simulink model "EM_SS_Model"  (R2017b)
settings: Solver=VariableStepAuto  StartTime=0.0  StopTime=10.0  RelTol=1e-3
undefined symbols (not defined in the file): Ax, Bx, Cx, Dx, u_0, x_0
settings Model: Creator=lasse  LastModifiedBy=lasse

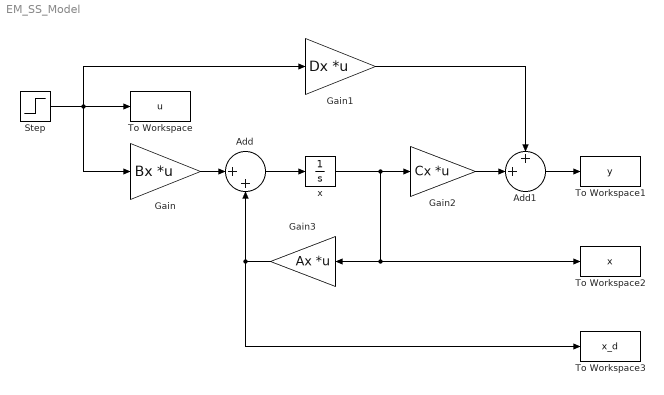
== system EM_SS_Model ==
  Add : Sum  Inputs=|++
  Add1 : Sum  Inputs=++|
  Gain : Gain  Gain=Bx  Multiplication=Matrix(K*u) (u vector)
  Gain1 : Gain  Gain=Dx  Multiplication=Matrix(K*u) (u vector)
  Gain2 : Gain  Gain=Cx  Multiplication=Matrix(K*u) (u vector)
  Gain3 : Gain  Gain=Ax  Multiplication=Matrix(K*u) (u vector)
  Step : Step  After=u_0  SampleTime=0
  To Workspace : ToWorkspace  VariableName=u  SaveFormat=Structure With Time  SampleTime=-1
  To Workspace1 : ToWorkspace  VariableName=y  SaveFormat=Structure With Time  SampleTime=-1
  To Workspace2 : ToWorkspace  VariableName=x  SaveFormat=Structure With Time  SampleTime=-1
  To Workspace3 : ToWorkspace  VariableName=x_d  SaveFormat=Structure With Time  SampleTime=-1
  x : Integrator  InitialCondition=x_0
  wires:
  Step/1 -> To Workspace/1, Gain/1, Gain1/1
  x/1 -> Gain2/1, Gain3/1, To Workspace2/1
  Gain/1 -> Add/1
  Add/1 -> x/1
  Gain3/1 -> To Workspace3/1, Add/2
  Gain2/1 -> Add1/2
  Gain1/1 -> Add1/1
  Add1/1 -> To Workspace1/1
